simulink model "sim03"  (R2020a)
settings: Solver=VariableStepAuto  StartTime=0.0  StopTime=10.0  RelTol=1e-3
values from neighbouring files (symbols this model uses):
  czas_skoku = 40    [lab01.m]    (also in sprawozdanie.m = 60)
  duTkz = 0    [lab01.m]    (also in sprawozdanie.m)
  duTzew = 0    [lab01.m]    (also in sprawozdanie.m)
  L1 = Ko*Ks + M2*Ks    [lab01.m]    (also in skrypt.m = M2*Cp*Pp*fp)
  L2 = M2*Cp*Pp*fp    [lab01.m]    (also in skrypt.m = Ko*Ks + M2*Ks)
  L3 = M1*Ks+Ks*Ko+Ks*Cp*Pp*fp    [lab01.m]    (also in skrypt.m = Cp*Pp*fp*(Cp*Pp*fp+Ko))
  L4 = Cp*Pp*fp*(Cp*Pp*fp+Ko)    [lab01.m]    (also in skrypt.m = M1*Ks+Ks*Ko+Ks*Cp*Pp*fp)
  M = [Cv1*Cv2,(Cv1+Cv2)*(Cp*Pp*fp+Ks+Ko),(Cp*Pp*fp+Ks+Ko)^2-Ko*(Cp*Pp*fp+Ko)]    [lab01.m]    (also in skrypt.m)
  Tw10 = ((Ko+Ks+Cp*Pp*fp)*(Cp*Pp*Tkz*fp+Ks*Tzew)+Ko*Ks*Tzew)/((Cp*Pp*fp+Ks+Ko)^2-Ko*(Ko+Cp*Pp*fp))    [lab01.m]    (also in sprawozdanie.m)
  Tw20 = (Tw10*(Ko+Cp*Pp*fp)+Ks*Tzew)/(Ko+Ks+Cp*Pp*fp)    [lab01.m]    (also in sprawozdanie.m)
settings Model: Creator=jakub  LastModifiedBy=jakub

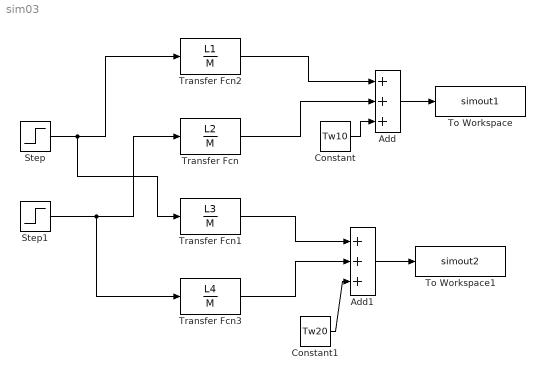
== system sim03 ==
  Add : Sum  Inputs=+++
  Add1 : Sum  Inputs=+++
  Constant : Constant  Value=Tw10
  Constant1 : Constant  Value=Tw20
  Step : Step  Time=czas_skoku  After=duTzew  SampleTime=0
  Step1 : Step  Time=czas_skoku  After=duTkz  SampleTime=0
  To Workspace : ToWorkspace  VariableName=simout1  SampleTime=-1
  To Workspace1 : ToWorkspace  VariableName=simout2  SampleTime=-1
  Transfer Fcn : TransferFcn  Numerator=L2  Denominator=M
  Transfer Fcn1 : TransferFcn  Numerator=L3  Denominator=M
  Transfer Fcn2 : TransferFcn  Numerator=L1  Denominator=M
  Transfer Fcn3 : TransferFcn  Numerator=L4  Denominator=M
  wires:
  Transfer Fcn/1 -> Add/2
  Constant1/1 -> Add1/3
  Transfer Fcn3/1 -> Add1/2
  Add/1 -> To Workspace/1
  Transfer Fcn1/1 -> Add1/1
  Transfer Fcn2/1 -> Add/1
  Constant/1 -> Add/3
  Step/1 -> Transfer Fcn1/1, Transfer Fcn2/1
  Step1/1 -> Transfer Fcn3/1, Transfer Fcn/1
  Add1/1 -> To Workspace1/1
